simulink model "HW1_MooreV2"  (R2017a)
settings: Solver=VariableStepAuto  StartTime=0.0  StopTime=inf  RelTol=1e-3
settings Model: Creator=avise  LastModifiedBy=nauga

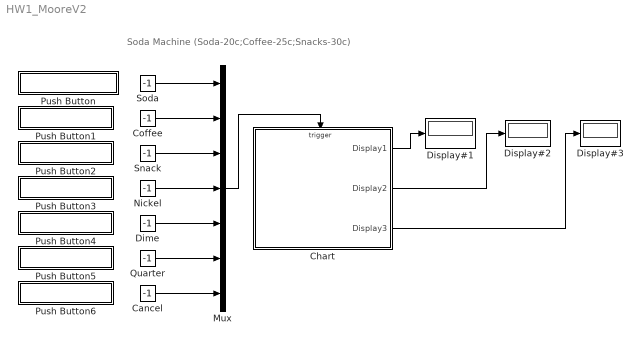
== system HW1_MooreV2 ==
  note: Soda Machine
      | (Soda-20c;Coffee-25c;Snacks-30c)
  Cancel : Constant  Value=-1
  Chart : Stateflow chart  TreatAsAtomicUnit=on
  Coffee : Constant  Value=-1
  Dime : Constant  Value=-1
  Display#1 : Display
  Display#2 : Display
  Display#3 : Display
  Mux : Mux  Inputs=7
  Nickel : Constant  Value=-1
  Push Button : Subsystem  DialogController=hmiCreateDDGDialog  IsWebBlock=on  mask(MWDashboardBlock){webBlockId=664f21db-061d-45c4-a5ed-301e6e3db717, webBlockType=pushbutton, ShowInLibBrwoser=on, ShowInitialText=on, HMISrcModelName=HW1_MooreV2}
      mask prompts: webBlockId "WebBlock Id"; webBlockType "WebBlock Type"; HMISrcModelName "Source Model"
      mask help: SimulinkHMI:dialogs:PushButtonDialogDesc
      mask Help: helpview([docroot '/mapfiles/simulink.map'], 'hmi_push_button')
      mask Display:
      | model = bdroot(gcb);
      | if strcmp(get_param(model,'BlockDiagramType'), 'library')
      |     image([(matlabroot) '/toolbox/simulink/hmi/icons/PushButton.png']);
      | end
  Push Button1 : Subsystem  DialogController=hmiCreateDDGDialog  IsWebBlock=on  mask(MWDashboardBlock){webBlockId=369ec6e0-de46-472e-8dd1-8918505b40b8, webBlockType=pushbutton, ShowInLibBrwoser=on, ShowInitialText=on, HMISrcModelName=HW1_MooreV2}
      mask prompts: webBlockId "WebBlock Id"; webBlockType "WebBlock Type"; HMISrcModelName "Source Model"
      mask help: SimulinkHMI:dialogs:PushButtonDialogDesc
      mask Help: helpview([docroot '/mapfiles/simulink.map'], 'hmi_push_button')
      mask Display:
      | model = bdroot(gcb);
      | if strcmp(get_param(model,'BlockDiagramType'), 'library')
      |     image([(matlabroot) '/toolbox/simulink/hmi/icons/PushButton.png']);
      | end
  Push Button2 : Subsystem  DialogController=hmiCreateDDGDialog  IsWebBlock=on  mask(MWDashboardBlock){webBlockId=437ecff1-f85d-43e6-a183-e5cb8b815949, webBlockType=pushbutton, ShowInLibBrwoser=on, ShowInitialText=on, HMISrcModelName=HW1_MooreV2}
      mask prompts: webBlockId "WebBlock Id"; webBlockType "WebBlock Type"; HMISrcModelName "Source Model"
      mask help: SimulinkHMI:dialogs:PushButtonDialogDesc
      mask Help: helpview([docroot '/mapfiles/simulink.map'], 'hmi_push_button')
      mask Display:
      | model = bdroot(gcb);
      | if strcmp(get_param(model,'BlockDiagramType'), 'library')
      |     image([(matlabroot) '/toolbox/simulink/hmi/icons/PushButton.png']);
      | end
  Push Button3 : Subsystem  DialogController=hmiCreateDDGDialog  IsWebBlock=on  mask(MWDashboardBlock){webBlockId=f2e822cd-a8a7-4ab8-9e8e-7b39c5c413d8, webBlockType=pushbutton, ShowInLibBrwoser=on, ShowInitialText=on, HMISrcModelName=HW1_MooreV2}
      mask prompts: webBlockId "WebBlock Id"; webBlockType "WebBlock Type"; HMISrcModelName "Source Model"
      mask help: SimulinkHMI:dialogs:PushButtonDialogDesc
      mask Help: helpview([docroot '/mapfiles/simulink.map'], 'hmi_push_button')
      mask Display:
      | model = bdroot(gcb);
      | if strcmp(get_param(model,'BlockDiagramType'), 'library')
      |     image([(matlabroot) '/toolbox/simulink/hmi/icons/PushButton.png']);
      | end
  Push Button4 : Subsystem  DialogController=hmiCreateDDGDialog  IsWebBlock=on  mask(MWDashboardBlock){webBlockId=f0c8a644-454f-4bf4-a778-a88d9125c533, webBlockType=pushbutton, ShowInLibBrwoser=on, ShowInitialText=on, HMISrcModelName=HW1_MooreV2}
      mask prompts: webBlockId "WebBlock Id"; webBlockType "WebBlock Type"; HMISrcModelName "Source Model"
      mask help: SimulinkHMI:dialogs:PushButtonDialogDesc
      mask Help: helpview([docroot '/mapfiles/simulink.map'], 'hmi_push_button')
      mask Display:
      | model = bdroot(gcb);
      | if strcmp(get_param(model,'BlockDiagramType'), 'library')
      |     image([(matlabroot) '/toolbox/simulink/hmi/icons/PushButton.png']);
      | end
  Push Button5 : Subsystem  DialogController=hmiCreateDDGDialog  IsWebBlock=on  mask(MWDashboardBlock){webBlockId=21d649ba-39b7-4048-9903-c8ade3fb44d4, webBlockType=pushbutton, ShowInLibBrwoser=on, ShowInitialText=on, HMISrcModelName=HW1_MooreV2}
      mask prompts: webBlockId "WebBlock Id"; webBlockType "WebBlock Type"; HMISrcModelName "Source Model"
      mask help: SimulinkHMI:dialogs:PushButtonDialogDesc
      mask Help: helpview([docroot '/mapfiles/simulink.map'], 'hmi_push_button')
      mask Display:
      | model = bdroot(gcb);
      | if strcmp(get_param(model,'BlockDiagramType'), 'library')
      |     image([(matlabroot) '/toolbox/simulink/hmi/icons/PushButton.png']);
      | end
  Push Button6 : Subsystem  DialogController=hmiCreateDDGDialog  IsWebBlock=on  mask(MWDashboardBlock){webBlockId=33373d40-ddda-4141-b1fc-f71dcaba8225, webBlockType=pushbutton, ShowInLibBrwoser=on, ShowInitialText=on, HMISrcModelName=HW1_MooreV2}
      mask prompts: webBlockId "WebBlock Id"; webBlockType "WebBlock Type"; HMISrcModelName "Source Model"
      mask help: SimulinkHMI:dialogs:PushButtonDialogDesc
      mask Help: helpview([docroot '/mapfiles/simulink.map'], 'hmi_push_button')
      mask Display:
      | model = bdroot(gcb);
      | if strcmp(get_param(model,'BlockDiagramType'), 'library')
      |     image([(matlabroot) '/toolbox/simulink/hmi/icons/PushButton.png']);
      | end
  Quarter : Constant  Value=-1
  Snack : Constant  Value=-1
  Soda : Constant  Value=-1
  wires:
  Cancel/1 -> Mux/7
  Snack/1 -> Mux/3
  Soda/1 -> Mux/1
  Coffee/1 -> Mux/2
  Chart/1(Display1) -> Display#1/1
  Mux/1 -> Chart/Trigger
  Quarter/1 -> Mux/6
  Dime/1 -> Mux/5
  Nickel/1 -> Mux/4
  Chart/2(Display2) -> Display#2/1
  Chart/3(Display3) -> Display#3/1

== system HW1_MooreV2/Push Button ==

== system HW1_MooreV2/Push Button1 ==

== system HW1_MooreV2/Push Button2 ==

== system HW1_MooreV2/Push Button3 ==

== system HW1_MooreV2/Push Button4 ==

== system HW1_MooreV2/Push Button5 ==

== system HW1_MooreV2/Push Button6 ==

== stateflow chart HW1_MooreV2/Chart ==
  state SodaCycle
    state TwentyCents
      state s1
        en:Display1=0;Display2=0;Display3=10;Reset
      state s2
        en:Display1=0;Display2=0;Display3=0;Reset
      state s3
        en:Display1=0;Display2=0;Display3=15;Reset
      state s4
        en:Display1=0;Display2=0;Display3=20;Reset
      state s5
        en:Display1=0;Display2=0;Display3=5;Reset
    state FiveCents
      state s1
        en:Display2=5;
      state err1
        en:Display1=9;
      (default) -> SodaCycle.FiveCents.s1
      FiveCents -> SodaCycle.FiveCents.err1 [order 1] : Coffee|Snack
    state TenCents
      state s1
        en:Display1=1;Display2=10
      state err1
        en:Display1=9;
      (default) -> SodaCycle.TenCents.s1
      TenCents -> SodaCycle.TenCents.err1 [order 1] : Coffee|Snack
    state FifteenCents
      state s1
        en:Display1=1;Display2=15;
      state err1
        en:Display1=9;
      (default) -> SodaCycle.FifteenCents.s1
      FifteenCents -> SodaCycle.FifteenCents.err1 [order 1] : Coffee|Snack
    FiveCents -> SodaCycle.TwentyCents.s1 [order 3] : Quarter
    FiveCents -> FifteenCents [order 2] : Dime
    TenCents -> SodaCycle.TwentyCents.s1 [order 4] : Cancel
    FiveCents -> TenCents [order 1] : Nickel
    TenCents -> FifteenCents [order 1] : Nickel
    FifteenCents -> SodaCycle.TwentyCents.s4 [order 1] : Nickel
    TenCents -> SodaCycle.TwentyCents.s2 [order 2] : Dime
    TenCents -> SodaCycle.TwentyCents.s3 [order 3] : Quarter
    FifteenCents -> SodaCycle.TwentyCents.s4 [order 3] : Quarter
    FifteenCents -> SodaCycle.TwentyCents.s3 [order 4] : Cancel
    FifteenCents -> SodaCycle.TwentyCents.s5 [order 2] : Dime
    FiveCents -> SodaCycle.TwentyCents.s5 [order 4] : Cancel
  state Wait
    state s3
      en:Display3=25;
    state Default
    state s1
      en:Display3=5;
    state s2
      en:Display3=10;
    Wait -> Wait.s3 [order 2] : Quarter
    (default) -> Default
    Wait -> Wait.s1 [order 3] : Nickel
    Wait -> Wait.s2 [order 1] : Dime
  state Soda
    %20c
    en:
    Display1=1;
    Display3=-1;
  state CoffeeCycle
    state Five
      state s1
        en:Display2=5;
      state err1
        en:Display1=9;
      (default) -> CoffeeCycle.Five.s1
      CoffeeCycle.Five -> CoffeeCycle.Five.err1 [order 1] : Soda|Snack
    state Ten
      state s1
        en:Display1=2;Display2=10;
      state err1
        en:Display1=9;
      (default) -> CoffeeCycle.Ten.s1
      CoffeeCycle.Ten -> CoffeeCycle.Ten.err1 [order 1] : Soda|Snack
    state Fifteen
      state s1
        en:Display1=2;Display2=15;
      state err1
        en:Display1=9;
      (default) -> CoffeeCycle.Fifteen.s1
      CoffeeCycle.Fifteen -> CoffeeCycle.Fifteen.err1 [order 1] : Soda|Snack
    state Twenty
      state s1
        en:Display1=2;Display2=20;
      state err1
        en:Display1=9;
      (default) -> CoffeeCycle.Twenty.s1
      CoffeeCycle.Twenty -> CoffeeCycle.Twenty.err1 [order 1] : Soda|Snack
    state TwentyFive
      state s1
        en:Display1=0;Display2=0;Display3=10;Reset
      state s2
        en:Display1=0;Display2=0;Display3=0;Reset
      state s3
        en:Display1=0;Display2=0;Display3=15;Reset
      state s4
        en:Display1=0;Display2=0;Display3=20;Reset
      state s5
        en:Display1=0;Display2=0;Display3=5;Reset
    CoffeeCycle.Fifteen -> CoffeeCycle.TwentyFive.s3 [order 3] : Quarter
    CoffeeCycle.Five -> CoffeeCycle.Fifteen [order 3] : Dime
    CoffeeCycle.Ten -> CoffeeCycle.Twenty [order 3] : Dime
    CoffeeCycle.Five -> CoffeeCycle.Ten [order 2] : Nickel
    CoffeeCycle.Five -> CoffeeCycle.TwentyFive.s5 [order 4] : Quarter
    CoffeeCycle.Ten -> CoffeeCycle.TwentyFive.s1 [order 4] : Quarter
    CoffeeCycle.Fifteen -> CoffeeCycle.Twenty [order 1] : Nickel
    CoffeeCycle.Ten -> CoffeeCycle.TwentyFive.s1 [order 1] : Cancel
    CoffeeCycle.Ten -> CoffeeCycle.Fifteen [order 2] : Nickel
    CoffeeCycle.Fifteen -> CoffeeCycle.TwentyFive.s2 [order 2] : Dime
    CoffeeCycle.Twenty -> CoffeeCycle.TwentyFive.s2 [order 1] : Nickel
    CoffeeCycle.Twenty -> CoffeeCycle.TwentyFive.s5 [order 2] : Dime
    CoffeeCycle.Fifteen -> CoffeeCycle.TwentyFive.s3 [order 4] : Cancel
    CoffeeCycle.Twenty -> CoffeeCycle.TwentyFive.s4 [order 3] : Quarter
    CoffeeCycle.Twenty -> CoffeeCycle.TwentyFive.s4 [order 4] : Cancel
    CoffeeCycle.Five -> CoffeeCycle.TwentyFive.s5 [order 1] : Cancel
  state Coffee
    %25c
    en:
    Display1=2;
    Display3=-1;
  state SnackCycle
    state Five
      state s1
        en:Display2=5;
      state err1
        en:Display1=9;
      (default) -> SnackCycle.Five.s1
      SnackCycle.Five -> SnackCycle.Five.err1 [order 1] : Soda|Coffee
    state Ten
      state s1
        en:Display1=3;Display2=10;
      state err1
        en:Display1=9;
      (default) -> SnackCycle.Ten.s1
      SnackCycle.Ten -> SnackCycle.Ten.err1 [order 1] : Soda|Coffee
    state Fifteen
      state s1
        en:Display1=3;Display2=15;
      state err1
        en:Display1=9;
      (default) -> SnackCycle.Fifteen.s1
      SnackCycle.Fifteen -> SnackCycle.Fifteen.err1 [order 1] : Soda|Coffee
    state Twenty
      state s1
        en:Display1=3;Display2=20;
      state err1
        en:Display1=9;
      (default) -> SnackCycle.Twenty.s1
      SnackCycle.Twenty -> SnackCycle.Twenty.err1 [order 1] : Soda|Coffee
    state TwentyFive
      state s1
        en:Display1=3;Display2=25;
      state err1
        en:Display1=9;
      (default) -> SnackCycle.TwentyFive.s1
      SnackCycle.TwentyFive -> SnackCycle.TwentyFive.err1 [order 1] : Soda|Coffee
    state Thirty
      state s1
        en:Display1=0;Display2=0;Display3=10;Reset
      state s2
        en:Display1=0;Display2=0;Display3=0;Reset
      state s3
        en:Display1=0;Display2=0;Display3=15;Reset
      state s4
        en:Display1=0;Display2=0;Display3=20;Reset
      state s5
        en:Display1=0;Display2=0;Display3=5;Reset
      state s6
        en:Display1=0;Display2=0;Display3=25;Reset
    SnackCycle.Twenty -> SnackCycle.Thirty.s3 [order 4] : Quarter
    SnackCycle.Ten -> SnackCycle.Thirty.s5 [order 3] : Quarter
    SnackCycle.Five -> SnackCycle.Fifteen [order 2] : Dime
    SnackCycle.Fifteen -> SnackCycle.TwentyFive [order 2] : Dime
    SnackCycle.Ten -> SnackCycle.Thirty.s1 [order 4] : Cancel
    SnackCycle.Five -> SnackCycle.Ten [order 1] : Nickel
    SnackCycle.Fifteen -> SnackCycle.Thirty.s1 [order 3] : Quarter
    SnackCycle.Ten -> SnackCycle.Twenty [order 2] : Dime
    SnackCycle.Fifteen -> SnackCycle.Twenty [order 1] : Nickel
    SnackCycle.Ten -> SnackCycle.Fifteen [order 1] : Nickel
    SnackCycle.Twenty -> SnackCycle.Thirty.s2 [order 3] : Dime
    SnackCycle.Twenty -> SnackCycle.TwentyFive [order 2] : Nickel
    SnackCycle.Five -> SnackCycle.Thirty.s2 [order 3] : Quarter
    SnackCycle.TwentyFive -> SnackCycle.Thirty.s2 [order 2] : Nickel
    SnackCycle.TwentyFive -> SnackCycle.Thirty.s5 [order 3] : Dime
    SnackCycle.Fifteen -> SnackCycle.Thirty.s3 [order 4] : Cancel
    SnackCycle.TwentyFive -> SnackCycle.Thirty.s4 [order 4] : Quarter
    SnackCycle.Twenty -> SnackCycle.Thirty.s4 [order 1] : Cancel
    SnackCycle.Five -> SnackCycle.Thirty.s5 [order 4] : Cancel
    SnackCycle.TwentyFive -> s6 [order 1] : Cancel
  state Snack
    %30c
    en:
    Display1=3;
    Display3=-1;
  (default) -> Wait
  Soda -> FiveCents [order 1] : Nickel
  Wait -> Soda [order 3] : Soda
  Wait -> Wait [order 2] : Cancel
  Soda -> TenCents [order 2] : Dime
  TwentyCents -> Wait : Reset
  CoffeeCycle.TwentyFive -> Wait : Reset
  Soda -> SodaCycle.TwentyCents.s5 [order 3] : Quarter
  Wait -> Snack [order 4] : Snack
  Thirty -> Wait : Reset
  Wait -> Coffee [order 1] : Coffee
  Coffee -> CoffeeCycle.Five [order 1] : Nickel
  Coffee -> CoffeeCycle.Ten [order 2] : Dime
  Coffee -> CoffeeCycle.TwentyFive.s2 [order 3] : Quarter
  Snack -> SnackCycle.Five [order 1] : Nickel
  Snack -> SnackCycle.Ten [order 2] : Dime
  Snack -> SnackCycle.TwentyFive [order 3] : Quarter
  data: Display1 output =0; Display2 output =0; Display3 output =-1
  events: Soda input EITHER_EDGE_EVENT; Coffee input EITHER_EDGE_EVENT; Snack input EITHER_EDGE_EVENT; Nickel input RISING_EDGE_EVENT; Dime input RISING_EDGE_EVENT; Quarter input RISING_EDGE_EVENT; Cancel input EITHER_EDGE_EVENT; Reset local FUNCTION_CALL_EVENT
